simulink model "BTL_vitri_vantoc"  (R2018a)
settings: Solver=VariableStepAuto  StartTime=0.0  StopTime=15  RelTol=1e-3
values from neighbouring files (symbols this model uses):
  km = 0.5    [Parameters.m]    (also in Parameters.mat; parametersAcc.m; parametersPos.m; parametersVel.m)
  KP = 5    [Parameters.m]    (also in Parameters.mat; parametersAcc.m = 26; parametersPos.m; parametersVel.m)
  kTP = 1    [Parameters.m]    (also in Parameters.mat; parametersAcc.m; parametersPos.m; parametersVel.m)
  kTV = 1    [Parameters.m]    (also in Parameters.mat; parametersAcc.m; parametersVel.m)
  KV = 10    [Parameters.m]    (also in Parameters.mat; parametersAcc.m = 12; parametersVel.m)
  Tm = 0    [Parameters.m]    (also in Parameters.mat = 5; parametersAcc.m = 0.025; parametersPos.m = 0.025; parametersVel.m = 0.025)
  TV = 0    [Parameters.m]    (also in Parameters.mat = 5; parametersAcc.m = 0.025; parametersVel.m = 0.025)
libraries: simulink x1
settings Model: Creator=Nguyen Mai  LastModifiedBy=Nguyen Mai

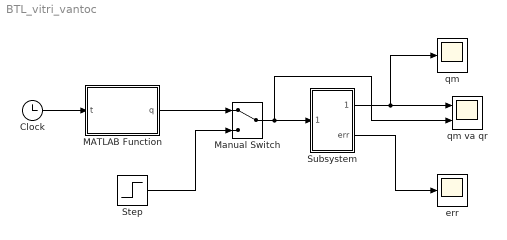
== system BTL_vitri_vantoc ==
  Clock : Clock
  MATLAB Function : MATLAB Function  TreatAsAtomicUnit=on
  Manual Switch : ManualSwitch
  Step : Step  SampleTime=0
  Subsystem : Subsystem
  err : Scope
  "qm " : Scope
  qm va qr : Scope  NumInputPorts=2
  wires:
  MATLAB Function/1(q) -> Manual Switch/1
  Step/1 -> Manual Switch/2
  Clock/1 -> MATLAB Function/1(t)
  Manual Switch/1 -> qm va qr/2, Subsystem/1(In1)
  Subsystem/2(err) -> err/1
  Subsystem/1(qm) -> "qm "/1, qm va qr/1

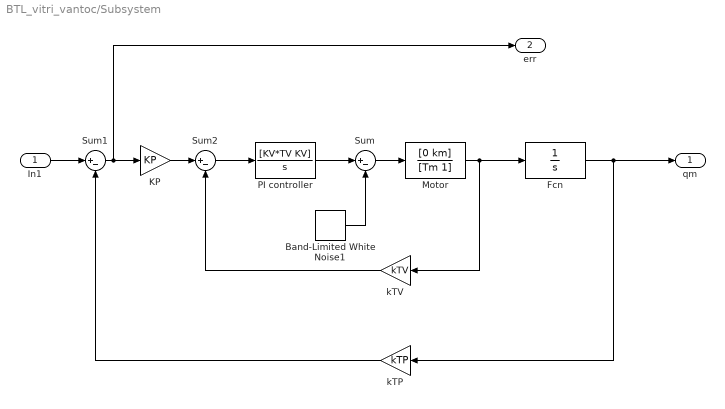
== system BTL_vitri_vantoc/Subsystem ==
  In1 : Inport
  Band-Limited White Noise1 : simulink/Sources/Band-Limited White Noise  Cov=[0.1]  Ts=0.1  seed=[23341]
  Fcn : TransferFcn  Denominator=[1 0]
  KP : Gain  Gain=KP
  Motor : TransferFcn  Numerator=[0 km]  Denominator=[Tm 1]
  PI controller : TransferFcn  Numerator=[KV*TV KV]  Denominator=[1 0]
  Sum : Sum  Inputs=|+-
  Sum1 : Sum  Inputs=|+-
  Sum2 : Sum  Inputs=|+-
  kTP : Gain  Gain=kTP
  kTV : Gain  Gain=kTV
  qm : Outport
  err : Outport  Port=2
  wires:
  In1/1 -> Sum1/1
  KP/1 -> Sum2/1
  Sum2/1 -> PI controller/1
  Sum1/1 -> KP/1, err/1
  Band-Limited White Noise1/1 -> Sum/2
  kTV/1 -> Sum2/2
  PI controller/1 -> Sum/1
  kTP/1 -> Sum1/2
  Motor/1 -> kTV/1, Fcn/1
  Fcn/1 -> qm/1, kTP/1
  Sum/1 -> Motor/1

== matlab function BTL_vitri_vantoc/MATLAB Function ==
  data: t input; q output
function q = fcn(t)
t0=0;
tf=50;
tc=10;
if t<tc
q=40+(43/40)*t^2;
else
if t<tf-tc
q=-(135/2)+(43/2)*t;
else
q=900-(43/40)*(50-t)^2;
end
end
